simulink model "LTRTenzo6Dof"  (R2017a)
settings: Solver=ode45  StartTime=0.0  StopTime=10  RelTol=1e-3  EnableMultiTasking=on
values from neighbouring files (symbols this model uses):
  A0 = tenzo_min_nominale.a    [HTenzoV10.m]    (also in HTenzoV11.m; HTenzoV12.m; HTenzoV13.m; HTenzoV14.m)
  amplitudeNoise = 2    [HTenzoV10.m]    (also in HTenzoV11.m; HTenzoV12.m; HTenzoV13.m; HTenzoV14.m)
  amplitudePertIn = 200    [HTenzoV13.m]    (also in HTenzoV14.m; HTenzoV20.m; HTenzoV21.m)
  amplitudePertOut = 0    [HTenzoV10.m]    (also in HTenzoV11.m; HTenzoV12.m; HTenzoV13.m; HTenzoV14.m)
  B0 = tenzo_min_nominale.b    [HTenzoV10.m]    (also in HTenzoV11.m; HTenzoV12.m; HTenzoV13.m; HTenzoV14.m)
  C0 = tenzo_min_nominale.c    [HTenzoV10.m]    (also in HTenzoV11.m; HTenzoV12.m; HTenzoV13.m; HTenzoV14.m)
  cstPertIn = 0    [HTenzoV10.m]    (also in HTenzoV11.m; HTenzoV12.m; HTenzoV13.m; HTenzoV14.m)
  cstPertOut = 0    [HTenzoV10.m]    (also in HTenzoV11.m; HTenzoV12.m; HTenzoV13.m; HTenzoV14.m)
  D0 = tenzo_min_nominale.d    [HTenzoV10.m]    (also in HTenzoV11.m; HTenzoV12.m; HTenzoV13.m; HTenzoV14.m)
  dcgX = ureal('dcgX',0.288,'Range',[0.25 0.30])    [HTenzoV1.m]    (also in HTenzoV10.m = ureal('dcgX',0.288,'Range',[0.12 0.40]); HTenzoV11.m = ureal('dcgX',0.288,'Range',[0.22 0.40]); HTenzoV12.m = ureal('dcgX',0.288,'Range',[0.22 0.40]); HTenzoV13.m = ureal('dcgX',0.288,'Range',[0.22 0.40]))
  dcgY = ureal('dcgY',0.288,'Range',[0.25 0.30])    [HTenzoV1.m]    (also in HTenzoV10.m = ureal('dcgY',0.288,'Range',[0.12 0.40]); HTenzoV11.m = ureal('dcgY',0.288,'Range',[0.22 0.40]); HTenzoV12.m = ureal('dcgY',0.288,'Range',[0.22 0.40]); HTenzoV13.m = ureal('dcgY',0.288,'Range',[0.22 0.40]))
  g = 9.81    [HTenzoV1.m]    (also in HTenzoV10.m; HTenzoV11.m; HTenzoV12.m; HTenzoV13.m)
  If = ureal('If',-0.3559,'Range',[-0.4000 -0.1559])    [HTenzoV1.m]    (also in HTenzoV10.m; HTenzoV11.m; HTenzoV12.m; HTenzoV13.m)
  KAoss = tenzo_min_nominale.a-L_3*tenzo_min_nominale.c    [HTenzoV12.m]    (also in HTenzoV13.m; HTenzoV14.m; HTenzoV20.m; HTenzoV21.m)
  KBossw = [tenzo_min_nominale.b-L_3*D L_3]    [HTenzoV12.m]    (also in HTenzoV13.m; HTenzoV14.m; HTenzoV20.m; HTenzoV21.m)
  KCoss = eye(size(Aoss,1))    [HTenzoV12.m]    (also in HTenzoV13.m; HTenzoV14.m; HTenzoV20.m; HTenzoV21.m)
  KDoss = zeros(size(Aoss,1),poss)    [HTenzoV12.m]    (also in HTenzoV13.m; HTenzoV14.m; HTenzoV20.m; HTenzoV21.m)
  Kopt = Kopt_3    [HTenzoV10.m]    (also in HTenzoV11.m; HTenzoV12.m; HTenzoV13.m; HTenzoV14.m)
  Kt = ct*rho*rp^4*pi()    [HTenzoV1.m]    (also in HTenzoV10.m; HTenzoV11.m; HTenzoV12.m; HTenzoV13.m)
  Ktm = Km/Kt    [HTenzoV1.m]    (also in HTenzoV10.m; HTenzoV11.m; HTenzoV12.m; HTenzoV13.m)
  mq = ureal('mq',1.150,'Range',[0.820 1.4224])    [HTenzoV1.m]    (also in HTenzoV10.m = ureal('mq',1.30,'Range',[0.020 2.0]); HTenzoV11.m = ureal('mq',1.30,'Range',[0.800 2.0]); HTenzoV12.m = ureal('mq',1.30,'Range',[0.800 2.0]); HTenzoV13.m = ureal('mq',1.30,'Range',[0.800 2.0]))
  omegaNoise = 370    [HTenzoV10.m]    (also in HTenzoV11.m; HTenzoV12.m; HTenzoV13.m; HTenzoV14.m)
  omegaPertIN = 6    [HTenzoV10.m]    (also in HTenzoV11.m; HTenzoV12.m; HTenzoV13.m; HTenzoV14.m)
  omegaPertOut = 0.1    [HTenzoV10.m]    (also in HTenzoV11.m; HTenzoV12.m; HTenzoV13.m; HTenzoV14.m)
  randomAmpNoise = 1    [HTenzoV10.m]    (also in HTenzoV11.m; HTenzoV12.m; HTenzoV13.m; HTenzoV14.m)
  tc = 100    [HTenzoV14.m]    (also in HTenzoV20.m; HTenzoV21.m)
undefined symbols (not defined in the file or in its folder): magnitude, sigbuilder_block
libraries: simulink_extras x2, aerolibobsolete x1
settings Model: SimulationMode=rapid-accelerator  Creator=danilo  LastModifiedBy=userk
settings DataIOCC: LimitDataPoints=on  SaveFormat=Array
settings OptimizationCC: ExpressionDepthLimit=2147483647  LifeSpan=inf
settings DebuggingCC: UnderspecifiedInitializationDetection=Classic  MergeDetectMultiDrivingBlocksExec=none  SolverPrmCheckMsg=warning  FcnCallInpInsideContextMsg=warning  AllowSymbolicDim=off  StateNameClashWarn=warning  SFUnexpectedBacktrackingDiag=warning  SFNoUnconditionalDefaultTransitionDiag=warning  SFExecutionAtInitializationDiag=none
settings HardwareCC: ProdBitPerPointer=32  ProdBitPerSizeT=32  ProdBitPerPtrDiffT=32  ProdLargestAtomicFloat=None  ProdIntDivRoundTo=Undefined  ProdEndianess=Unspecified  ProdWordSize=32  ProdHWDeviceType=32-bit Generic
settings ModelReferenceCC: PropagateSignalLabelsOutOfModel=off
settings GRTTargetCC: TargetLangStandard=C89/C90 (ANSI)  GeneratePreprocessorConditionals=Disable all  CombineOutputUpdateFcns=off  GRTInterface=on
settings ConfigComp: CovMetricSettings=dw  CovHtmlReporting=on  CovSaveCumulativeToWorkspaceVar=on  CovSaveSingleToWorkspaceVar=on  CovExternalEMLEnable=off

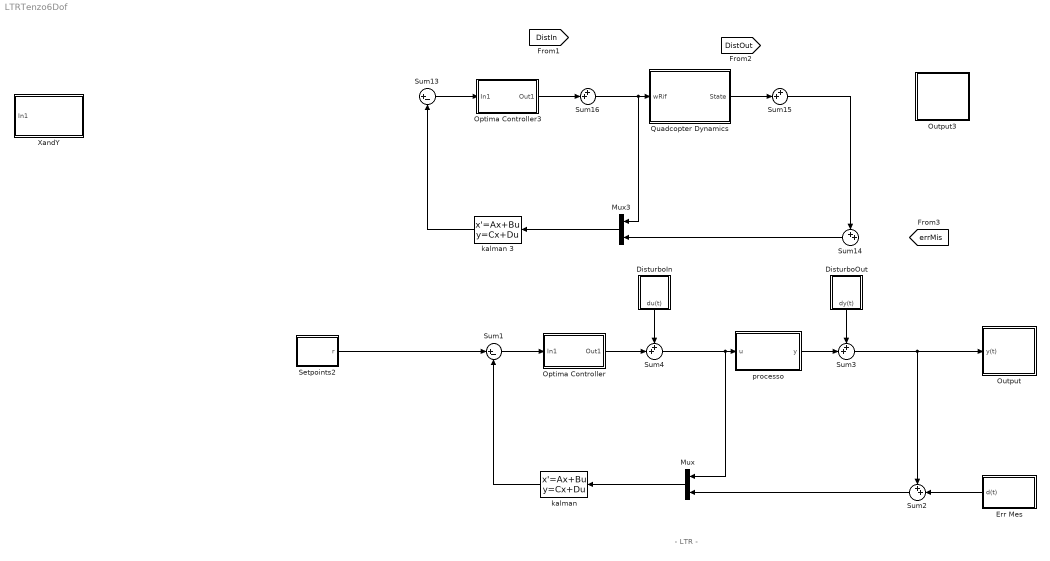
== system LTRTenzo6Dof ==
  note: - LTR -
  " kalman " : StateSpace  A=KAoss  B=KBossw  C=KCoss  D=KDoss  X0=0
  " kalman 3" : StateSpace  A=KAoss  B=KBossw  C=KCoss  D=KDoss  X0=0
  DisturboIn : Subsystem
  DisturboOut : Subsystem
  Err Mes : Subsystem
  Mux : Mux  Inputs=2
  Mux3 : Mux  Inputs=2
  Optima Controller : Subsystem
  Optima Controller3 : Subsystem
  Output : Subsystem
  Output3 : Subsystem
  Quadcopter Dynamics : Subsystem
  Setpoints2 : Subsystem
  Sum1 : Sum  Inputs=|+-
  Sum13 : Sum  Inputs=|+-
  Sum{2..4,14..16} (6 alike) : Sum  Inputs=++|
  XandY : Subsystem
  processo : Subsystem
  wires:
  Sum2/1 -> Mux/2
  processo/1(y) -> Sum3/2
  DisturboIn/1(du(t)) -> Sum4/1
  Sum3/1 -> Sum2/1, Output/1(y(t))
  DisturboOut/1("dy(t) ") -> Sum3/1
  Sum1/1 -> Optima Controller/1(In1)
  Optima Controller/1(Out1) -> Sum4/2
  Mux/1 -> " kalman "/1
  " kalman "/1 -> Sum1/2
  Sum4/1 -> Mux/1, processo/1(u)
  Setpoints2/1(r) -> Sum1/1
  Err Mes/1("  d(t)") -> Sum2/2
  Sum14/1 -> Mux3/2
  Quadcopter Dynamics/1(State) -> Sum15/2
  Sum15/1 -> Sum14/1
  Sum13/1 -> Optima Controller3/1(In1)
  Optima Controller3/1(Out1) -> Sum16/2
  Mux3/1 -> " kalman 3"/1
  " kalman 3"/1 -> Sum13/2
  Sum16/1 -> Mux3/1, Quadcopter Dynamics/1(wRif)

== system LTRTenzo6Dof/DisturboIn ==
  ErrIn : Subsystem
  Mux : Mux  Inputs=[1 1 1 1]
  dist : Scope
  du(t) : Outport
  tag scope: DistIn=global
  wires:
  Mux/1 -> dist/1, [DistIn], du(t)/1
  ErrIn/1(Out1) -> Mux/4, Mux/3, Mux/2, Mux/1

== system LTRTenzo6Dof/DisturboOut ==
  ErrOut : Subsystem
  Mux : Mux  Inputs=[1 1 1 1]
  dist : Scope
  "dy(t) " : Outport
  tag scope: DistOut=global
  wires:
  ErrOut/1(Out1) -> Mux/4, Mux/3, Mux/2, Mux/1
  Mux/1 -> "dy(t) "/1, [DistOut], dist/1

== system LTRTenzo6Dof/Err Mes ==
  Filtered random noise + sin : Subsystem
  Mux : Mux  Inputs=[1 1 1 1]
  NoiseScope : Scope
  "  d(t)" : Outport
  tag scope: errMis=global
  wires:
  Mux/1 -> [errMis], NoiseScope/1, "  d(t)"/1
  Filtered random noise + sin/1(n(t)) -> Mux/4, Mux/3, Mux/2, Mux/1

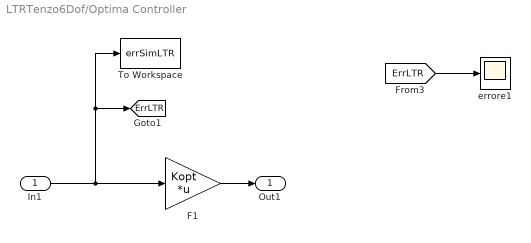
== system LTRTenzo6Dof/Optima Controller ==
  In1 : Inport
  F1 : Gain  Gain=Kopt  Multiplication=Matrix(K*u) (u vector)
  To Workspace : ToWorkspace  VariableName=errSimLTR  SaveFormat=Structure  SampleTime=-1
  errore1 : Scope
  Out1 : Outport
  tag scope: ErrLTR=global
  wires:
  In1/1 -> F1/1, To Workspace/1, [ErrLTR]
  F1/1 -> Out1/1
  [ErrLTR] -> errore1/1

== system LTRTenzo6Dof/Optima Controller3 ==
  In1 : Inport
  F1 : Gain  Gain=Kopt  Multiplication=Matrix(K*u) (u vector)
  To Workspace : ToWorkspace  VariableName=errSim  SaveFormat=Structure  SampleTime=-1
  errore1 : Scope
  Out1 : Outport
  tag scope: ErrNL=global
  wires:
  In1/1 -> F1/1, To Workspace/1, [ErrNL]
  F1/1 -> Out1/1
  [ErrNL] -> errore1/1

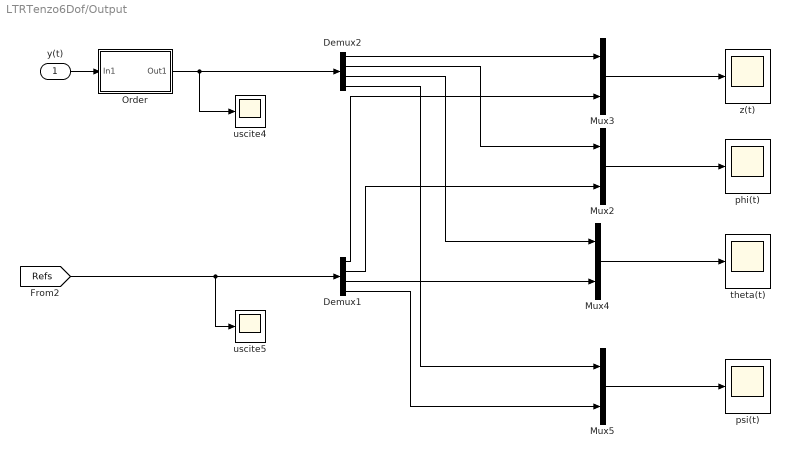
== system LTRTenzo6Dof/Output ==
  y(t) : Inport
  Demux1 : Demux
  Demux2 : Demux
  Mux{2..5} (4 alike) : Mux  Inputs=2
  "Order " : Subsystem
  phi(t) : Scope
  psi(t) : Scope
  theta(t) : Scope
  uscite4 : Scope
  uscite5 : Scope
  z(t) : Scope
  wires:
  [Refs] -> Demux1/1, uscite5/1
  Demux1/1 -> Mux3/2
  Mux2/1 -> phi(t)/1
  Demux2/2 -> Mux2/1
  Mux3/1 -> z(t)/1
  Demux2/1 -> Mux3/1
  Mux4/1 -> theta(t)/1
  Demux2/3 -> Mux4/1
  Mux5/1 -> psi(t)/1
  Demux2/4 -> Mux5/1
  Demux1/2 -> Mux2/2
  Demux1/3 -> Mux4/2
  Demux1/4 -> Mux5/2
  "Order "/1(Out1) -> Demux2/1, uscite4/1
  y(t)/1 -> "Order "/1(In1)

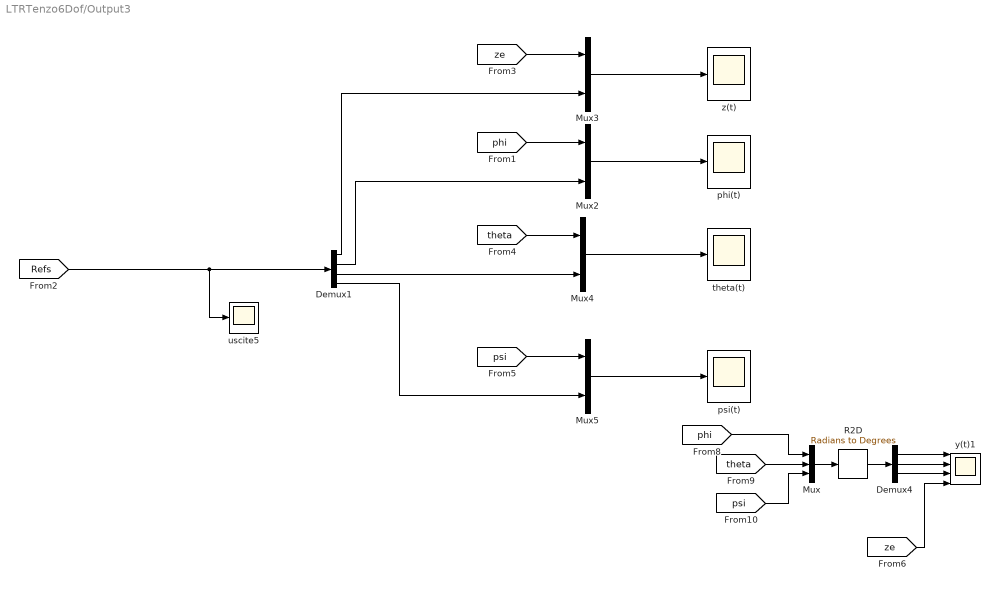
== system LTRTenzo6Dof/Output3 ==
  Demux1 : Demux
  Demux4 : Demux  Outputs=3
  Mux : Mux  Inputs=3
  Mux{2..5} (4 alike) : Mux  Inputs=2
  R2D : simulink_extras/Transformations/Radians to Degrees
  phi(t) : Scope
  psi(t) : Scope
  theta(t) : Scope
  uscite5 : Scope
  y(t)1 : Scope  NumInputPorts=4
  z(t) : Scope
  wires:
  [Refs] -> Demux1/1, uscite5/1
  Demux1/1 -> Mux3/2
  Mux2/1 -> phi(t)/1
  [phi] -> Mux2/1
  Mux3/1 -> z(t)/1
  [ze] -> Mux3/1
  Mux4/1 -> theta(t)/1
  [theta] -> Mux4/1
  Mux5/1 -> psi(t)/1
  [psi] -> Mux5/1
  Demux1/2 -> Mux2/2
  Demux1/3 -> Mux4/2
  Demux1/4 -> Mux5/2
  [ze] -> y(t)1/4
  R2D/1 -> Demux4/1
  [phi] -> Mux/1
  [theta] -> Mux/2
  [psi] -> Mux/3
  Mux/1 -> R2D/1
  Demux4/1 -> y(t)1/1
  Demux4/2 -> y(t)1/2
  Demux4/3 -> y(t)1/3

== system LTRTenzo6Dof/Quadcopter Dynamics ==
  wRif : Inport
  Motors(t) : Subsystem
  Sum1 : Sum  Inputs=|++
  Tenzo NL : Subsystem
  WtoTreal : Subsystem
  "u(t) " : Scope
  State : Outport
  wires:
  WtoTreal/1(U(t)) -> Tenzo NL/1(Yinertial)
  Tenzo NL/1(State) -> State/1
  wRif/1 -> Sum1/1
  Sum1/1 -> "u(t) "/1, WtoTreal/1(w(t))

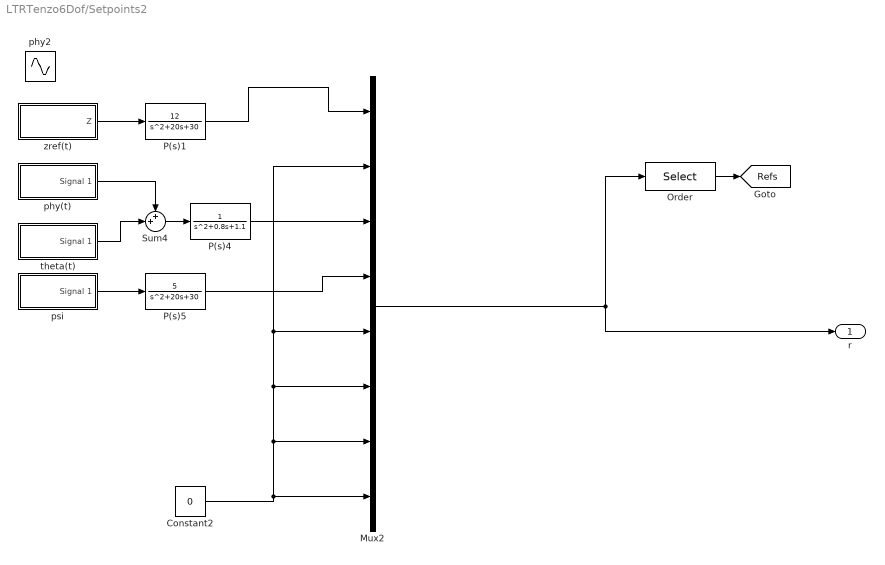
== system LTRTenzo6Dof/Setpoints2 ==
  Constant2 : Constant  Value=0
  Mux2 : Mux  Inputs=[1 1 1 1 1 1 1 1]
  Order : Selector  InputPortWidth=8  IndexOptions=Index vector (dialog)  Indices=[1,3,4,5]  OutputSizes=1
  P(s)1 : TransferFcn  Numerator=12  Denominator=[1 20 30]
  P(s)4 : TransferFcn  Numerator=1  Denominator=[1 0.8 1.1]
  P(s)5 : TransferFcn  Numerator=5  Denominator=[1 20 30]
  Sum4 : Sum  Inputs=++|
  phy(t) : Subsystem  Tag=STV Subsys  LoadFcn=sigbuilder_block('load');  StartFcn=sigbuilder_block('start');  StopFcn=sigbuilder_block('stop');  ClipboardFcn=sigbuilder_block('clipboard');  mask(Sigbuilder block){tuvar=[0:10]}
      mask help: Simulink:masks:SigbuilderBlock_MD
      mask init:
      | if ~strcmp(get_param(bdroot(gcbh),'SimulationStatus'),'stopped') tuvar = sigbuilder_block('maskInit'); end
      settings: CopyFcn=sigbuilder_block('copy');  DeleteFcn=sigbuilder_block('delete');  ModelCloseFcn=sigbuilder_block('modelClose');  PreSaveFcn=sigbuilder_block('preSave');  PauseFcn=sigbuilder_block('pause');  ContinueFcn=sigbuilder_block('continue');  NameChangeFcn=sigbuilder_block('namechange');  OpenFcn=sigbuilder_block('open',[341.6 120.8 550.4 400 ]);  CloseFcn=sigbuilder_block('close');
      mask Display: plot(0, 0, 100, 100,[2, 2, 32, 32, 2], [68, 8, 8, 68, 68],[32, 2], [38, 38], [32, 19, 2],[53, 60, 44], [32, 17, 17, 2],[16, 16, 31, 31]);txt = getActiveGroup(gcbh);text(2, 100, txt,'verticalAlignment', 'top');
  phy2 : Sin  Amplitude=10  Frequency=0.2  SampleTime=0
  "psi " : Subsystem  Tag=STV Subsys  LoadFcn=sigbuilder_block('load');  StartFcn=sigbuilder_block('start');  StopFcn=sigbuilder_block('stop');  ClipboardFcn=sigbuilder_block('clipboard');  mask(Sigbuilder block){tuvar=[0:10]}
      mask help: Simulink:masks:SigbuilderBlock_MD
      mask init:
      | if ~strcmp(get_param(bdroot(gcbh),'SimulationStatus'),'stopped') tuvar = sigbuilder_block('maskInit'); end
      settings: CopyFcn=sigbuilder_block('copy');  DeleteFcn=sigbuilder_block('delete');  ModelCloseFcn=sigbuilder_block('modelClose');  PreSaveFcn=sigbuilder_block('preSave');  PauseFcn=sigbuilder_block('pause');  ContinueFcn=sigbuilder_block('continue');  NameChangeFcn=sigbuilder_block('namechange');  OpenFcn=sigbuilder_block('open',[341.6 120.8 550.4 400 ]);  CloseFcn=sigbuilder_block('close');
      mask Display: plot(0, 0, 100, 100,[2, 2, 32, 32, 2], [68, 8, 8, 68, 68],[32, 2], [38, 38], [32, 19, 2],[53, 60, 44], [32, 17, 17, 2],[16, 16, 31, 31]);txt = getActiveGroup(gcbh);text(2, 100, txt,'verticalAlignment', 'top');
  theta(t) : Subsystem  Tag=STV Subsys  LoadFcn=sigbuilder_block('load');  StartFcn=sigbuilder_block('start');  StopFcn=sigbuilder_block('stop');  ClipboardFcn=sigbuilder_block('clipboard');  mask(Sigbuilder block){tuvar=[0:10]}
      mask help: Simulink:masks:SigbuilderBlock_MD
      mask init:
      | if ~strcmp(get_param(bdroot(gcbh),'SimulationStatus'),'stopped') tuvar = sigbuilder_block('maskInit'); end
      settings: CopyFcn=sigbuilder_block('copy');  DeleteFcn=sigbuilder_block('delete');  ModelCloseFcn=sigbuilder_block('modelClose');  PreSaveFcn=sigbuilder_block('preSave');  PauseFcn=sigbuilder_block('pause');  ContinueFcn=sigbuilder_block('continue');  NameChangeFcn=sigbuilder_block('namechange');  OpenFcn=sigbuilder_block('open',[341.6 120.8 550.4 400 ]);  CloseFcn=sigbuilder_block('close');
      mask Display: plot(0, 0, 100, 100,[2, 2, 32, 32, 2], [68, 8, 8, 68, 68],[32, 2], [38, 38], [32, 19, 2],[53, 60, 44], [32, 17, 17, 2],[16, 16, 31, 31]);txt = getActiveGroup(gcbh);text(2, 100, txt,'verticalAlignment', 'top');
  zref(t) : Subsystem  Tag=STV Subsys  LoadFcn=sigbuilder_block('load');  StartFcn=sigbuilder_block('start');  StopFcn=sigbuilder_block('stop');  ClipboardFcn=sigbuilder_block('clipboard');  mask(Sigbuilder block){tuvar=[0:10]}
      mask help: Simulink:masks:SigbuilderBlock_MD
      mask init:
      | if ~strcmp(get_param(bdroot(gcbh),'SimulationStatus'),'stopped') tuvar = sigbuilder_block('maskInit'); end
      settings: CopyFcn=sigbuilder_block('copy');  DeleteFcn=sigbuilder_block('delete');  ModelCloseFcn=sigbuilder_block('modelClose');  PreSaveFcn=sigbuilder_block('preSave');  PauseFcn=sigbuilder_block('pause');  ContinueFcn=sigbuilder_block('continue');  NameChangeFcn=sigbuilder_block('namechange');  OpenFcn=sigbuilder_block('open',[341.6 120.8 550.4 400 ]);  CloseFcn=sigbuilder_block('close');
      mask Display: plot(0, 0, 100, 100,[2, 2, 32, 32, 2], [68, 8, 8, 68, 68],[32, 2], [38, 38], [32, 19, 2],[53, 60, 44], [32, 17, 17, 2],[16, 16, 31, 31]);txt = getActiveGroup(gcbh);text(2, 100, txt,'verticalAlignment', 'top');
  r : Outport
  tag scope: Refs=global
  wires:
  theta(t)/1(Signal 1) -> Sum4/2
  phy(t)/1(Signal 1) -> Sum4/1
  Sum4/1 -> P(s)4/1
  P(s)4/1 -> Mux2/3
  P(s)1/1 -> Mux2/1
  "psi "/1(Signal 1) -> P(s)5/1
  Constant2/1 -> Mux2/8, Mux2/7, Mux2/6, Mux2/2, Mux2/5
  zref(t)/1(Z) -> P(s)1/1
  Mux2/1 -> r/1, Order/1
  Order/1 -> [Refs]
  P(s)5/1 -> Mux2/4

== system LTRTenzo6Dof/XandY ==
  In1 : Inport
  C : MATLAB Function  TreatAsAtomicUnit=on
  Output1 : Subsystem
  Selector : Subsystem
  tag scope: RefsNL=global
  wires:
  Selector/1(Out1) -> [RefsNL]
  C/1(ymis) -> Output1/1(In1)
  In1/1 -> Selector/1(In1), C/1(X)

== system LTRTenzo6Dof/processo ==
  u : Inport
  Processo1 : StateSpace  A=A0  B=B0  C=C0  D=D0  X0=0
  Saturation2 : Saturate  UpperLimit=24000  LowerLimit=-24000
  "u(t) " : Scope
  y : Outport
  wires:
  Processo1/1 -> y/1
  u/1 -> "u(t) "/1, Processo1/1

== system LTRTenzo6Dof/DisturboIn/ErrIn ==
  Clock : Clock
  Constant : Constant  Value=0
  Switch : Switch  Threshold=5
  disturbo : Subsystem
  Out1 : Outport
  wires:
  Constant/1 -> Switch/3
  disturbo/1(d) -> Switch/1
  Switch/1 -> Out1/1  "DiturboStato"
  Clock/1 -> Switch/2

== system LTRTenzo6Dof/DisturboOut/ErrOut ==
  Clock : Clock
  Constant : Constant  Value=0
  Switch : Switch  Threshold=5
  disturbo : Subsystem
  Out1 : Outport
  wires:
  Clock/1 -> Switch/2
  Switch/1 -> Out1/1  "DiturboStato"
  disturbo/1(d) -> Switch/1
  Constant/1 -> Switch/3

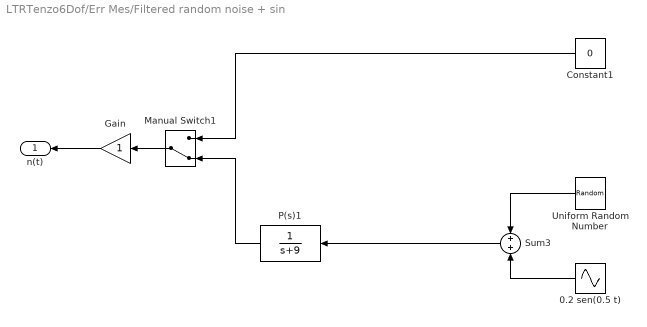
== system LTRTenzo6Dof/Err Mes/Filtered random noise + sin ==
  0.2 sen(0.5 t) : Sin  Amplitude=amplitudeNoise  Frequency=omegaNoise  Phase=1  SampleTime=0
  Constant1 : Constant  Value=0
  Gain : Gain
  Manual Switch1 : ManualSwitch  CurrentSetting=0
  P(s)1 : TransferFcn  Numerator=1  Denominator=[1 9]
  Sum3 : Sum
  Uniform Random Number : UniformRandomNumber  Minimum=-randomAmpNoise  Maximum=randomAmpNoise  SampleTime=0.1
  n(t) : Outport
  wires:
  Uniform Random Number/1 -> Sum3/1
  Constant1/1 -> Manual Switch1/1
  Sum3/1 -> P(s)1/1
  Gain/1 -> n(t)/1
  P(s)1/1 -> Manual Switch1/2
  Manual Switch1/1 -> Gain/1
  0.2 sen(0.5 t)/1 -> Sum3/2

== system LTRTenzo6Dof/Output/Order  ==
  In1 : Inport
  Demux3 : Demux
  Mux1 : Mux
  Out1 : Outport
  wires:
  Demux3/2 -> Mux1/3
  Demux3/1 -> Mux1/2
  In1/1 -> Demux3/1
  Mux1/1 -> Out1/1
  Demux3/4 -> Mux1/1
  Demux3/3 -> Mux1/4

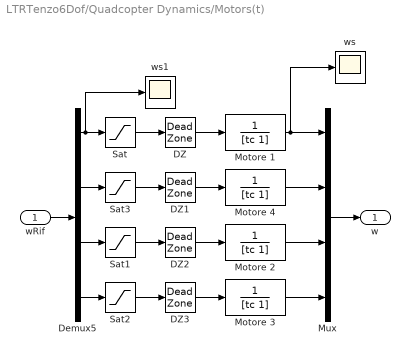
== system LTRTenzo6Dof/Quadcopter Dynamics/Motors(t) ==
  wRif : Inport
  DZ : DeadZone  LowerValue=0  UpperValue=10  SaturateOnIntegerOverflow=on
  DZ1 : DeadZone  LowerValue=0  UpperValue=300  SaturateOnIntegerOverflow=on
  DZ2 : DeadZone  LowerValue=0  UpperValue=300  SaturateOnIntegerOverflow=on
  DZ3 : DeadZone  LowerValue=0  UpperValue=300  SaturateOnIntegerOverflow=on
  Demux5 : Demux
  Motore {1..4} (4 alike) : TransferFcn  Denominator=[tc 1]
  Mux : Mux
  Sat{,1..3} (4 alike) : Saturate  UpperLimit=10000  LowerLimit=0
  ws : Scope
  ws1 : Scope
  w : Outport
  wires:
  Mux/1 -> w/1
  wRif/1 -> Demux5/1
  Motore 3/1 -> Mux/4
  Demux5/4 -> Sat2/1
  Motore 2/1 -> Mux/3
  Demux5/3 -> Sat1/1
  Motore 4/1 -> Mux/2
  Demux5/2 -> Sat3/1
  DZ1/1 -> Motore 4/1
  Sat3/1 -> DZ1/1
  DZ3/1 -> Motore 3/1
  Sat2/1 -> DZ3/1
  DZ2/1 -> Motore 2/1
  Sat1/1 -> DZ2/1
  Motore 1/1 -> Mux/1, ws/1
  DZ/1 -> Motore 1/1
  Sat/1 -> DZ/1
  Demux5/1 -> Sat/1, ws1/1

== system LTRTenzo6Dof/Quadcopter Dynamics/Tenzo NL ==
  Yinertial : Inport
  Quadcopter Dynamics : Subsystem
  TorquesForces : Subsystem
  State : Outport
  wires:
  Yinertial/1 -> TorquesForces/1(Inputs)
  TorquesForces/1(Forces) -> Quadcopter Dynamics/1(In1)
  TorquesForces/2("Torques ") -> Quadcopter Dynamics/2(In2)
  Quadcopter Dynamics/1(Out1) -> State/1

== system LTRTenzo6Dof/Quadcopter Dynamics/WtoTreal ==
  w(t) : Inport
  Demux : Demux
  Mixer : Subsystem
  Mux : Mux
  SquareGains : Subsystem
  U(t) : Outport
  wires:
  Mux/1 -> U(t)/1
  w(t)/1 -> Demux/1
  Mixer/1(Out1) -> Mux/1
  Mixer/2(Out2) -> Mux/2
  Mixer/3(Out3) -> Mux/3
  Mixer/4(Out4) -> Mux/4
  Demux/1 -> SquareGains/1(w1)
  Demux/2 -> SquareGains/2(w2)
  Demux/3 -> SquareGains/3(w3)
  Demux/4 -> SquareGains/4(w4)
  SquareGains/1(Out1) -> Mixer/1(In1)
  SquareGains/2(Out2) -> Mixer/2(In2)
  SquareGains/3(Out3) -> Mixer/3(In3)
  SquareGains/4(Out4) -> Mixer/4(In4)

== system LTRTenzo6Dof/Setpoints2/phy(t) ==
  Demux : Demux  Tag=STV Demux  Outputs=1
  FromWs : FromWorkspace  Tag=STV FromWs  VariableName=tuvar  SampleTime=0
      SigBuilderData=|
      | common.afterFinalStr = 'Extrapolate'
      | common.sampleTime = 0
      | dataSet.timeRange = [0 10]
      | dataSet.name = 'Group 1'
      | sbobj.Groups.Name = 'Group 1'
      | sbobj.Groups.Signals.Name = 'Signal 1'
      | sbobj.Groups.Signals.XData = [0 0.98 2 2 10]
      | sbobj.Groups.Signals.YData = [0 0 50 0 0]
  Signal 1 : Outport  Tag=STV Outport
  wires:
  Demux/1 -> Signal 1/1
  FromWs/1 -> Demux/1

== system LTRTenzo6Dof/Setpoints2/psi  ==
  Demux : Demux  Tag=STV Demux  Outputs=1
  FromWs : FromWorkspace  Tag=STV FromWs  VariableName=tuvar  SampleTime=0
      SigBuilderData=|
      | common.afterFinalStr = 'Extrapolate'
      | common.sampleTime = 0
      | dataSet.timeRange = [0 10]
      | dataSet.name = 'Group 1'
      | sbobj.Groups.Name = 'Group 1'
      | sbobj.Groups.Signals.Name = 'Signal 1'
      | sbobj.Groups.Signals.XData = [0 4.06 6.82 10]
      | sbobj.Groups.Signals.YData = [0 190 0 0]
  Signal 1 : Outport  Tag=STV Outport
  wires:
  Demux/1 -> Signal 1/1
  FromWs/1 -> Demux/1

== system LTRTenzo6Dof/Setpoints2/theta(t) ==
  Demux : Demux  Tag=STV Demux  Outputs=1
  FromWs : FromWorkspace  Tag=STV FromWs  VariableName=tuvar  SampleTime=0
      SigBuilderData=|
      | common.afterFinalStr = 'Extrapolate'
      | common.sampleTime = 0
      | dataSet.timeRange = [0 10]
      | dataSet.name = 'Group 1'
      | sbobj.Groups.Name = 'Group 1'
      | sbobj.Groups.Signals.Name = 'Signal 1'
      | sbobj.Groups.Signals.XData = [0 1 2.06 4.06 6.82 6.82 10]
      | sbobj.Groups.Signals.YData = [0 0 10 0 20 0 0]
  Signal 1 : Outport  Tag=STV Outport
  wires:
  Demux/1 -> Signal 1/1
  FromWs/1 -> Demux/1

== system LTRTenzo6Dof/Setpoints2/zref(t) ==
  Demux : Demux  Tag=STV Demux  Outputs=1
  FromWs : FromWorkspace  Tag=STV FromWs  VariableName=tuvar  SampleTime=0
      SigBuilderData=|
      | common.afterFinalStr = 'Extrapolate'
      | common.sampleTime = 0
      | dataSet.timeRange = [0 10]
      | dataSet.name = 'Group 1'
      | sbobj.Groups.Name = 'Group 1'
      | sbobj.Groups.Signals.Name = 'Z'
      | sbobj.Groups.Signals.XData = [0 1 2.06 4.06 6.82 10]
      | sbobj.Groups.Signals.YData = [0 0 10 10 0 0]
  Z : Outport  Tag=STV Outport
  wires:
  FromWs/1 -> Demux/1
  Demux/1 -> Z/1

== system LTRTenzo6Dof/XandY/Output1 ==
  In1 : Inport
  Demux3 : Demux
  Demux4 : Demux  Outputs=3
  Mux : Mux  Inputs=3
  R2D : simulink_extras/Transformations/Radians to Degrees
  y(t)1 : Scope  NumInputPorts=4
  wires:
  In1/1 -> Demux3/1
  Demux3/4 -> y(t)1/4
  R2D/1 -> Demux4/1
  Demux3/1 -> Mux/1
  Demux3/2 -> Mux/2
  Demux3/3 -> Mux/3
  Mux/1 -> R2D/1
  Demux4/1 -> y(t)1/1
  Demux4/2 -> y(t)1/2
  Demux4/3 -> y(t)1/3

== system LTRTenzo6Dof/XandY/Selector ==
  In1 : Inport
  Bus Creator : BusCreator  Inputs=5
  Demux : Demux  Outputs=12
  Out1 : Outport
  wires:
  In1/1 -> Demux/1
  Bus Creator/1 -> Out1/1
  Demux/1 -> Bus Creator/1
  Demux/2 -> Bus Creator/2
  Demux/9 -> Bus Creator/3
  Demux/10 -> Bus Creator/4
  Demux/11 -> Bus Creator/5

== system LTRTenzo6Dof/DisturboIn/ErrIn/disturbo ==
  Constant : Constant  Value=cstPertIn
  SineIn : Sin  Amplitude=amplitudePertIn  Frequency=omegaPertIN  SampleTime=0
  Sum2 : Sum  Inputs=|++
  d : Outport
  wires:
  Sum2/1 -> d/1
  Constant/1 -> Sum2/1
  SineIn/1 -> Sum2/2

== system LTRTenzo6Dof/DisturboOut/ErrOut/disturbo ==
  Constant : Constant  Value=cstPertOut
  SinOut : Sin  Amplitude=amplitudePertOut  Frequency=omegaPertOut  SampleTime=0
  Sum2 : Sum  Inputs=|++
  d : Outport
  wires:
  SinOut/1 -> Sum2/2
  Constant/1 -> Sum2/1
  Sum2/1 -> d/1

== system LTRTenzo6Dof/Quadcopter Dynamics/Tenzo NL/Quadcopter Dynamics ==
  note: 6dofDynamics
  In1 : Inport
  In2 : Inport  Port=2
  6DoF (Euler Angles) : aerolibobsolete/6DoF (Euler Angles)  units=Metric (MKS)  mtype=Fixed  rep=Euler Angles  xme_0=[0 0 0]  Vm_0=[0 0 0]  eul_0=[0 0 0]  pm_0=[0 0 0]  mass_0=mq.nominal  mass_e=0.5  mass_f=2.0  inertia=II.nominal  inertia_e=eye(3)  inertia_f=2*eye(3)  k_quat=1.0
      settings: SourceProductName=Aerospace Blockset  SourceProductBaseCode=AE
  order : Subsystem
  Out1 : Outport
  wires:
  In2/1 -> 6DoF (Euler Angles)/2
  In1/1 -> 6DoF (Euler Angles)/1
  6DoF (Euler Angles)/1 -> order/1(In1)
  6DoF (Euler Angles)/4 -> order/4(In4)
  6DoF (Euler Angles)/3 -> order/3(In3)
  6DoF (Euler Angles)/5 -> order/5(In5)
  6DoF (Euler Angles)/6 -> order/6(In6)
  6DoF (Euler Angles)/7 -> order/7(In7)
  6DoF (Euler Angles)/8 -> order/8(In8)
  6DoF (Euler Angles)/2 -> order/2(In2)
  order/1("y ") -> Out1/1

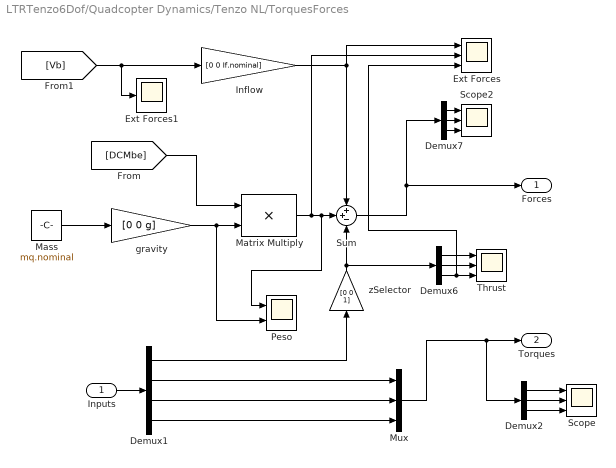
== system LTRTenzo6Dof/Quadcopter Dynamics/Tenzo NL/TorquesForces ==
  Inputs : Inport
  Demux1 : Demux
  Demux2 : Demux  Outputs=3
  Demux6 : Demux  Outputs=3
  Demux7 : Demux  Outputs=3
  Ext Forces : Scope  NumInputPorts=3
  Ext Forces1 : Scope
  Inflow : Gain  Gain=[0 0 If.nominal]
  Mass : Constant  Value=mq.nominal
  Matrix Multiply : Product
  Mux : Mux  Inputs=3
  Peso : Scope  NumInputPorts=2
  Scope : Scope  NumInputPorts=3
  Scope2 : Scope  NumInputPorts=3
  Sum : Sum  Inputs=++-
  Thrust : Scope  NumInputPorts=3
  gravity : Gain  Gain=[0 0 g]
  zSelector : Gain  Gain=[0 0 1]
  Forces : Outport
  "Torques " : Outport  Port=2
  wires:
  [DCMbe] -> Matrix Multiply/1
  Mass/1 -> gravity/1
  Matrix Multiply/1 -> Sum/2, Peso/1, Ext Forces/2
  gravity/1 -> Matrix Multiply/2, Peso/2
  [Vb] -> Inflow/1, Ext Forces1/1
  Inflow/1 -> Sum/1, Ext Forces/1
  Demux1/1 -> zSelector/1
  Demux1/2 -> Mux/1
  Demux1/3 -> Mux/2
  Demux1/4 -> Mux/3
  Sum/1 -> Forces/1, Demux7/1
  Mux/1 -> "Torques "/1, Demux2/1
  Demux2/1 -> Scope/1
  Inputs/1 -> Demux1/1
  Demux2/2 -> Scope/2
  Demux2/3 -> Scope/3
  Demux7/1 -> Scope2/1
  Demux7/2 -> Scope2/2
  Demux7/3 -> Scope2/3
  zSelector/1 -> Sum/3, Demux6/1
  Demux6/1 -> Thrust/1
  Demux6/2 -> Thrust/2
  Demux6/3 -> Thrust/3, Ext Forces/3

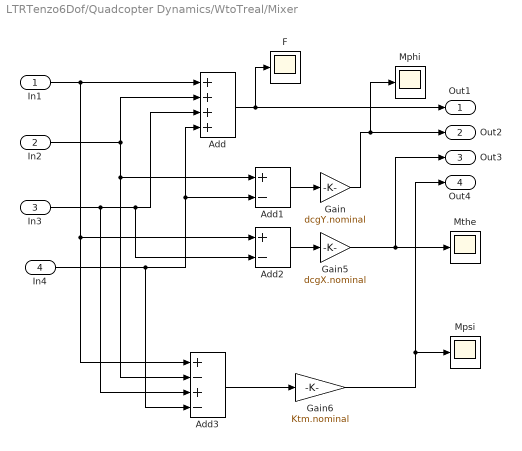
== system LTRTenzo6Dof/Quadcopter Dynamics/WtoTreal/Mixer ==
  In1 : Inport
  In2 : Inport  Port=2
  In3 : Inport  Port=3
  In4 : Inport  Port=4
  Add : Sum  Inputs=++++
  Add1 : Sum  Inputs=+-
  Add2 : Sum  Inputs=+-
  Add3 : Sum  Inputs=+-+-
  F : Scope
  Gain : Gain  Gain=dcgY.nominal
  Gain5 : Gain  Gain=dcgX.nominal
  Gain6 : Gain  Gain=Ktm.nominal
  Mphi : Scope
  Mpsi : Scope
  Mthe : Scope
  Out1 : Outport
  Out2 : Outport  Port=2
  Out3 : Outport  Port=3
  Out4 : Outport  Port=4
  wires:
  In1/1 -> Add/1, Add2/1, Add3/1
  In2/1 -> Add/2, Add1/1, Add3/2
  In3/1 -> Add/3, Add2/2, Add3/3
  In4/1 -> Add/4, Add1/2, Add3/4
  Add/1 -> Out1/1, F/1
  Add1/1 -> Gain/1
  Add2/1 -> Gain5/1
  Gain/1 -> Out2/1, Mphi/1
  Gain5/1 -> Out3/1, Mthe/1
  Add3/1 -> Gain6/1
  Gain6/1 -> Out4/1, Mpsi/1

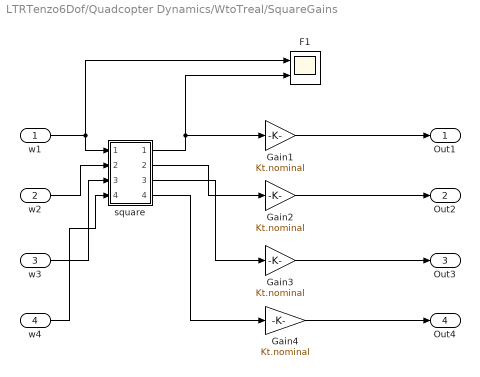
== system LTRTenzo6Dof/Quadcopter Dynamics/WtoTreal/SquareGains ==
  w1 : Inport
  w2 : Inport  Port=2
  w3 : Inport  Port=3
  w4 : Inport  Port=4
  F1 : Scope  NumInputPorts=2
  Gain{1..4} (4 alike) : Gain  Gain=Kt.nominal
  square : Subsystem
  Out1 : Outport
  Out2 : Outport  Port=2
  Out3 : Outport  Port=3
  Out4 : Outport  Port=4
  wires:
  Gain4/1 -> Out4/1
  Gain3/1 -> Out3/1
  Gain1/1 -> Out1/1
  w1/1 -> square/1(In1), F1/1
  Gain2/1 -> Out2/1
  square/1(Out1) -> Gain1/1, F1/2
  w2/1 -> square/2(In2)
  w3/1 -> square/3(In3)
  w4/1 -> square/4(In4)
  square/2(Out2) -> Gain2/1
  square/3(Out3) -> Gain3/1
  square/4(Out4) -> Gain4/1

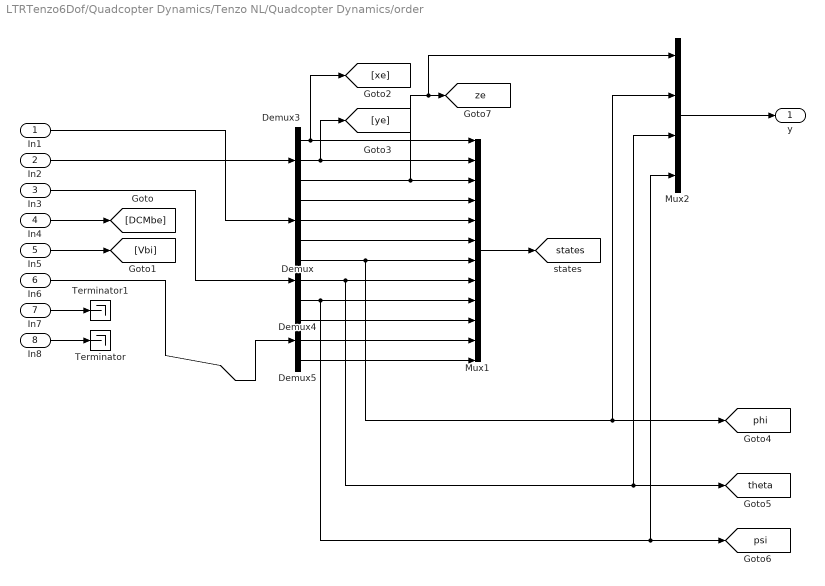
== system LTRTenzo6Dof/Quadcopter Dynamics/Tenzo NL/Quadcopter Dynamics/order ==
  In1 : Inport
  In2 : Inport  Port=2
  In3 : Inport  Port=3
  In4 : Inport  Port=4
  In5 : Inport  Port=5
  In6 : Inport  Port=6
  In7 : Inport  Port=7
  In8 : Inport  Port=8
  Demux{,3..5} (4 alike) : Demux  Outputs=3
  Mux1 : Mux  Inputs=12
  Mux2 : Mux
  Terminator : Terminator
  Terminator1 : Terminator
  "y " : Outport
  tag scope: phi=global, psi=global, states=global, theta=global, ze=global
  wires:
  In5/1 -> [Vbi]
  In4/1 -> [DCMbe]
  In1/1 -> Demux/1
  In2/1 -> Demux3/1
  Demux3/1 -> Mux1/1, [xe]
  Demux3/2 -> Mux1/2, [ye]
  Demux3/3 -> Mux1/3, Mux2/1, [ze]
  Demux/1 -> Mux1/4
  Demux/2 -> Mux1/5
  Demux/3 -> Mux1/6
  Demux4/1 -> Mux1/7, Mux2/2, [phi]
  Demux4/2 -> Mux1/8, Mux2/3, [theta]
  Demux4/3 -> Mux1/9, Mux2/4, [psi]
  Demux5/1 -> Mux1/10
  Demux5/2 -> Mux1/11
  Demux5/3 -> Mux1/12
  In8/1 -> Terminator/1
  In7/1 -> Terminator1/1
  In3/1 -> Demux4/1
  Mux1/1 -> [states]
  In6/1 -> Demux5/1
  Mux2/1 -> "y "/1

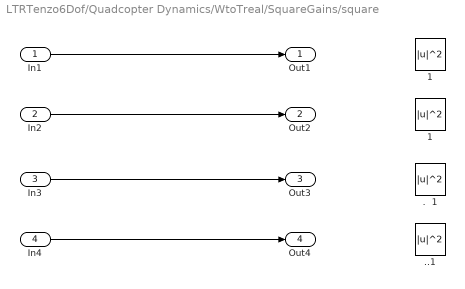
== system LTRTenzo6Dof/Quadcopter Dynamics/WtoTreal/SquareGains/square ==
  In1 : Inport
  In2 : Inport  Port=2
  In3 : Inport  Port=3
  In4 : Inport  Port=4
  " 1" : Math  Operator=magnitude^2  SaturateOnIntegerOverflow=on
  " 1" : Math  Operator=magnitude^2  SaturateOnIntegerOverflow=on
  .  1 : Math  Operator=magnitude^2  SaturateOnIntegerOverflow=on
  ..1 : Math  Operator=magnitude^2  SaturateOnIntegerOverflow=on
  Out1 : Outport
  Out2 : Outport  Port=2
  Out3 : Outport  Port=3
  Out4 : Outport  Port=4
  wires:
  In1/1 -> Out1/1
  In2/1 -> Out2/1
  In3/1 -> Out3/1
  In4/1 -> Out4/1

== matlab function LTRTenzo6Dof/XandY/C ==
  data: X input; ymis output
function ymis = fcn(X)
%#codegen

Cmis = [0 0 0 0 0 0 1 0 0 0 0 0;
        0 0 0 0 0 0 0 1 0 0 0 0;
        0 0 0 0 0 0 0 0 1 0 0 0;
        0 0 1 0 0 0 0 0 0 0 0 0];
ymis = Cmis*X;
